simulink model "sim1"  (Simulink 7.7)
settings: Solver=ode45  StartTime=0.0  StopTime=3*pi  MaxStep=0.1  RelTol=1e-3
settings Model: Creator=qcg  LastModifiedBy=qcg

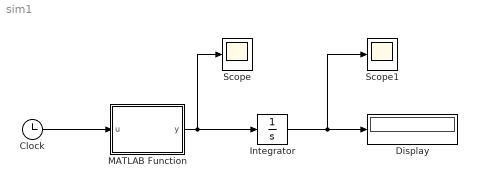
== system sim1 ==
  Clock : Clock
      settings: Decimation=10
  Display : Display
  Integrator : Integrator
  MATLAB Function : Stateflow chart  TreatAsAtomicUnit=on
  Scope : Scope
  Scope1 : Scope
  wires:
  Clock/1 -> MATLAB Function/1(u)
  MATLAB Function/1(y) -> Integrator/1, Scope/1
  Integrator/1 -> Display/1, Scope1/1

== matlab function MATLAB Function ==
  data: u input double; y output double
function y = fcn(u)
%#codegen

y = sqrt(cos(2*u)^2+sin(u)^2+1);
